simulink model "_simulinkSampledInput"  (R2017a)
settings: Solver=VariableStepAuto  StartTime=0.0  StopTime=30  RelTol=1e-3  EnableMultiTasking=on
undefined symbols (not defined in the file): A, B, C, D1, D2, h, K
settings Model: Creator=1513 IRON  LastModifiedBy=Rafael
settings OptimizationCC: LifeSpan=inf
settings DebuggingCC: SFUnexpectedBacktrackingDiag=warning  SFNoUnconditionalDefaultTransitionDiag=warning  SFExecutionAtInitializationDiag=none
settings GRTTargetCC: TargetLangStandard=C89/C90 (ANSI)  GeneratePreprocessorConditionals=Disable all
settings ConfigComp: CovMetricSettings=dw  CovHtmlReporting=on  CovSaveCumulativeToWorkspaceVar=on  CovSaveSingleToWorkspaceVar=on  CovExternalEMLEnable=off

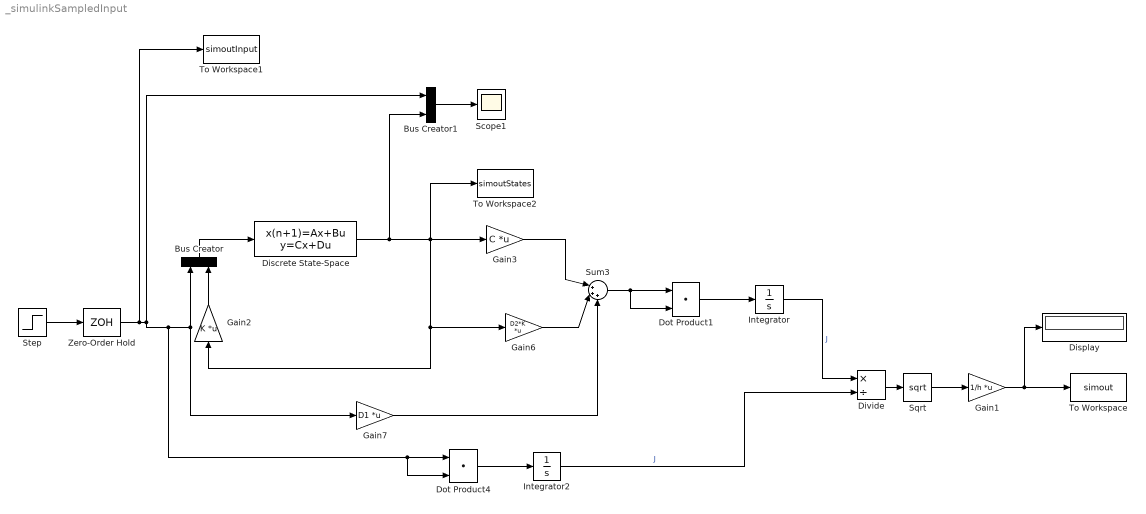
== system _simulinkSampledInput ==
  Bus Creator : BusCreator  Inputs=2
  Bus Creator1 : BusCreator  Inputs=2
  Discrete State-Space : DiscreteStateSpace  A=A  B=B  C=eye(size(A,1))  D=zeros(size(A,1),size(B,2))  X0=zeros(length(A),1)  SampleTime=h
  Display : Display
  Divide : Product  Inputs=*/
  Dot Product1 : DotProduct  InputSameDT=on  OutDataTypeStr=Inherit: Inherit via internal rule
  Dot Product4 : DotProduct  InputSameDT=on  OutDataTypeStr=Inherit: Inherit via internal rule
  Gain1 : Gain  Gain=1/h  Multiplication=Matrix(K*u)
  Gain2 : Gain  Gain=K  Multiplication=Matrix(K*u)
  Gain3 : Gain  Gain=C  Multiplication=Matrix(K*u)
  Gain6 : Gain  Gain=D2*K  Multiplication=Matrix(K*u)
  Gain7 : Gain  Gain=D1  Multiplication=Matrix(K*u)
  Integrator : Integrator
  Integrator2 : Integrator
  Scope1 : Scope
  Sqrt : Sqrt  SaturateOnIntegerOverflow=on
  Step : Step  Before=1  After=0  SampleTime=h
  Sum3 : Sum  Inputs=|+++
  To Workspace : ToWorkspace  VariableName=simout  SaveFormat=Timeseries  SampleTime=-1
  To Workspace1 : ToWorkspace  VariableName=simoutInput  SaveFormat=Timeseries  SampleTime=-1
  To Workspace2 : ToWorkspace  VariableName=simoutStates  SaveFormat=Timeseries  SampleTime=-1
  Zero-Order Hold : ZeroOrderHold  SampleTime=h
  wires:
  Integrator/1 -> Divide/1  "J"
  Gain2/1 -> Bus Creator/2
  Discrete State-Space/1 -> Bus Creator1/2, To Workspace2/1, Gain3/1, Gain6/1, Gain2/1
  Bus Creator/1 -> Discrete State-Space/1
  Step/1 -> Zero-Order Hold/1
  Gain3/1 -> Sum3/1
  Gain6/1 -> Sum3/2
  Sum3/1 -> Dot Product1/2, Dot Product1/1
  Gain7/1 -> Sum3/3
  Dot Product1/1 -> Integrator/1
  Zero-Order Hold/1 -> To Workspace1/1, Dot Product4/2, Dot Product4/1, Gain7/1, Bus Creator/1, Bus Creator1/1
  Dot Product4/1 -> Integrator2/1
  Integrator2/1 -> Divide/2  "J"
  Bus Creator1/1 -> Scope1/1
  Divide/1 -> Sqrt/1
  Sqrt/1 -> Gain1/1
  Gain1/1 -> Display/1, To Workspace/1
